simulink model "qweqwqwe"  (R2023a)
settings: Solver=VariableStepAuto  StartTime=0.0  StopTime=10  RelTol=1e-3
values from neighbouring files (symbols this model uses):
  J = [0.00031              0              -0.000004657 ... (first row only)    [paramm.m]
  K = 1256.637    [paramm.m]
  Km = 6.1028207267564559047121275317652e-7    (= 6.10282072676e-07)    [paramm.m]
  Kn = 6.1028207267564559047121275317652e-7    (= 6.10282072676e-07)    [paramm.m]
  l = 0.1125    [paramm.m]
  Phi_air_damping_constant = 0    [paramm.m]
  Psi_air_damping_constant = 0    [paramm.m]
  Tau = 0.001    [paramm.m]
  Theta_air_damping_constant = 0    [paramm.m]
undefined symbols (not defined in the file or in its folder): x_air_damping_ratio, y_air_damping_ratio, z_air_damping_ratio
libraries: dspsigops x15, slpidlib x6
(part 2 of 2)

== matlab function qweqwqwe/Subsystem4/Subsystem5/MATLAB Function1 ==
  data: u input; p_dot output; q_dot output; r_dot output
function [p_dot,q_dot,r_dot] = Rot(u)



%5p_dot =  [1 sin(Phi)*tan(Theta)   cos(Phi)*tan(Theta)]*u;
%q_dot =  [  0        cos(Phi)            -sin(Phi)]*u    ;
%r_dot =  [ 0  sin(Phi)*sec(Theta)   cos(Phi)*sec(Theta)]*u;

p_dot =  [1 0   0]*u;
q_dot =  [0  1   0]*u    ;
r_dot =  [ 0  0  1]*u;

 



end

== matlab function qweqwqwe/Subsystem4/Subsystem5/MATLAB Function2 ==
  data: u input; p_dot output; q_dot output; r_dot output
function [p_dot,q_dot,r_dot] = Rot(u)



%5p_dot =  [1 sin(Phi)*tan(Theta)   cos(Phi)*tan(Theta)]*u;
%q_dot =  [  0        cos(Phi)            -sin(Phi)]*u    ;
%r_dot =  [ 0  sin(Phi)*sec(Theta)   cos(Phi)*sec(Theta)]*u;

p_dot =  [1 0   0]*u;
q_dot =  [0  1   0]*u    ;
r_dot =  [ 0  0  1]*u;

 



end

== matlab function qweqwqwe/Subsystem4/Subsystem5/MATLAB Function ==
  data: Fz_b input; Phi input; Theta input; Psi input; u_dot output; v_dot output; r_dot output
function [u_dot,v_dot,r_dot] = fcn(Fz_b,Phi,Theta,Psi)
y =[(cos(Psi)*cos(Theta)) (cos(Psi)*sin(Theta)*sin(Phi)-sin(Psi)*cos(Phi)) (cos(Phi)*sin(Theta)*cos(Phi)+sin(Psi)*sin(Phi));
    (sin(Psi)*cos(Theta)) (sin(Psi)*sin(Theta)*sin(Phi)-cos(Psi)*cos(Phi)) (sin(Phi)*sin(Theta)*cos(Phi)-sin(Phi)*cos(Psi));
    (-sin(Theta)) (cos(Theta)*sin(Phi)) (cos(Theta)*cos(Phi))]*[0;0;Fz_b];

u_dot = y(1);
v_dot = y(2);
r_dot = y(3)+9.8;
end

== matlab function qweqwqwe/Subsystem4/Subsystem2/Subsystem2/Subsystem/MATLAB Function1 ==
  data: pp input; rp input; y output; J input
function y = fcn(pp,rp, J)

y = rp*(J(1,1)-J(3,3))-pp*(J(1,3));
end

== matlab function qweqwqwe/Subsystem4/Subsystem2/Subsystem2/Subsystem/MATLAB Function2 ==
  data: pq input; qr input; y output; J input
function y = fcn(pq,qr,J)

y = qr*(J(1,3))+pq*(J(2,2)-J(1,1));
end

== matlab function qweqwqwe/Subsystem4/Subsystem2/Subsystem2/Subsystem1/MATLAB Function ==
  data: cor_x input; Ang_acc_B output; cor_y input; cor_z input; M_B input; J input
function Ang_acc_B = fcn(cor_x, cor_y, cor_z, M_B, J)

Ang_acc_B = inv(J)*(M_B - [cor_x;cor_y;cor_z]);
end

== matlab function qweqwqwe/Subsystem4/Subsystem2/MATLAB Function3 ==
  data: x_air_damping_ratio input; z_air_damping_ratio input; u input; Phi input; u_air_damping output; Theta input
function u_air_damping = fcn(x_air_damping_ratio, z_air_damping_ratio, u,Phi, Theta)

u_air_damping = abs(z_air_damping_ratio*sin(Theta))+x_air_damping_ratio*cos(Phi)*u;

== matlab function qweqwqwe/Subsystem4/Subsystem2/MATLAB Function5 ==
  data: x_air_damping_constatn input; y_air_damping_constant input; z_air_damping_constant input; u input; Phi input; w_air_damping output; Theta input
function w_air_damping = fcn(x_air_damping_constatn,y_air_damping_constant, z_air_damping_constant, u,Phi, Theta)

w_air_damping =-( z_air_damping_constant*cos(Theta)+z_air_damping_constant*cos(Phi)+abs(x_air_damping_constatn*sin(Theta))+abs(y_air_damping_constant*sin(Phi)))*u;

== matlab function qweqwqwe/Subsystem4/Subsystem2/MATLAB Function7 ==
  data: Psi_air_damping_constant input; u input; q_dot_damped output; q_dot input
function q_dot_damped = fcn(Psi_air_damping_constant,u, q_dot)

q_dot_damped =q_dot-(Psi_air_damping_constant*u)/abs(q_dot)*q_dot;

== matlab function qweqwqwe/Subsystem4/Subsystem3/MATLAB Function ==
  data: O1 input; O2 input; O3 input; O4 input; Fz output; Mx output; My output; Mz output; Kn input; Km input; l input
function [Fz,Mx,My,Mz] = OM(O1, O2, O3, O4, Kn, Km ,l) 
Fz =  -Kn*(O1+O2+O3+O4)         ;
Mx=    l*Kn*0.707*(-O1+O2-O3+O4);
My=    l*Kn*0.707*(-O1+O2+O3-O4) ; 
Mz=   Km*(-O1-O2+O3+O4);
end

== matlab function qweqwqwe/Subsystem4/Subsystem2/MATLAB Function ==
  data: Fz_b input; Phi input; Theta input; Psi input; u_dot output; v_dot output; r_dot output
function [u_dot,v_dot,r_dot] = fcn(Fz_b,Phi,Theta,Psi)
y =[(cos(Psi)*cos(Theta)) (cos(Psi)*sin(Theta)*sin(Phi)-sin(Psi)*cos(Phi)) (cos(Phi)*sin(Theta)*cos(Phi)+sin(Psi)*sin(Phi));
    (sin(Psi)*cos(Theta)) (sin(Psi)*sin(Theta)*sin(Phi)-cos(Psi)*cos(Phi)) (sin(Phi)*sin(Theta)*cos(Phi)-sin(Phi)*cos(Psi));
    (-sin(Theta)) (cos(Theta)*sin(Phi)) (cos(Theta)*cos(Phi))]*[0;0;Fz_b];

u_dot = y(1);
v_dot = y(2);
r_dot = y(3)+9.8;
end

== matlab function qweqwqwe/Subsystem4/Subsystem4/MATLAB Function ==
  data: O1 input; O2 input; O3 input; O4 input; Fz output; Mx output; My output; Mz output; Kn input; Km input; l input
function [Fz,Mx,My,Mz] = OM(O1, O2, O3, O4, Kn, Km ,l) 
Fz =  -Kn*(O1+O2+O3+O4)         ;
Mx=    l*Kn*0.707*(-O1+O2-O3+O4);
My=    l*Kn*0.707*(-O1+O2+O3-O4) ; 
Mz=   -Km*(-O1-O2+O3+O4);
end

== matlab function qweqwqwe/Subsystem4/Subsystem1/MATLAB Function1 ==
  data: Mx input; M output; My input; Mz input
function M = fcn(Mx,My,Mz)

M = [Mx;    My  ;  Mz];
end

== matlab function qweqwqwe/Subsystem4/Subsystem2/MATLAB Function1 ==
  data: p input; skew output; q input; r input
function skew = sk(p,q,r)



skew = [0 -r q;
        r  0 -p;
        -q p  0];


 



end
